simulink model "PI_observador_ideal_jhon"  (R2021b)
settings: Solver=VariableStepAuto  StartTime=0.0  StopTime=8  RelTol=1e-3
values from neighbouring files (symbols this model uses):
  K = [9.27647435897 40.5008113553]    [ValidarpiO.mat]
  ki = 111.439929309    [ValidarpiO.mat]
libraries: cstblocks x5
settings Model: Creator=axelt  LastModifiedBy=parra
settings DebuggingCC: UnconnectedInputMsg=none  UnconnectedOutputMsg=none  UnconnectedLineMsg=none
settings ModelReferenceCC: EnableRefExpFcnMdlSchedulingChecks=off
settings RTWCC: DLArmComputeVersion=20.02.1

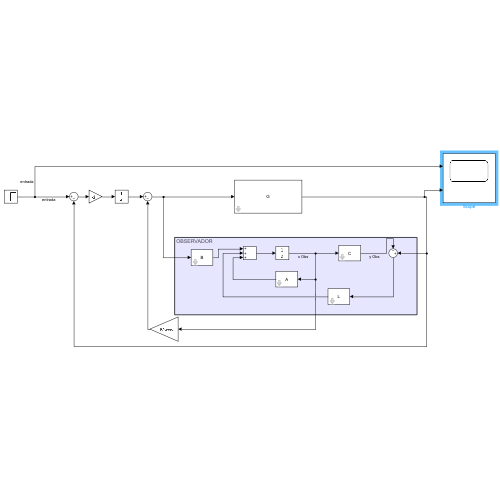
[thumbnail: Simulink's stored preview of the top-level diagram]
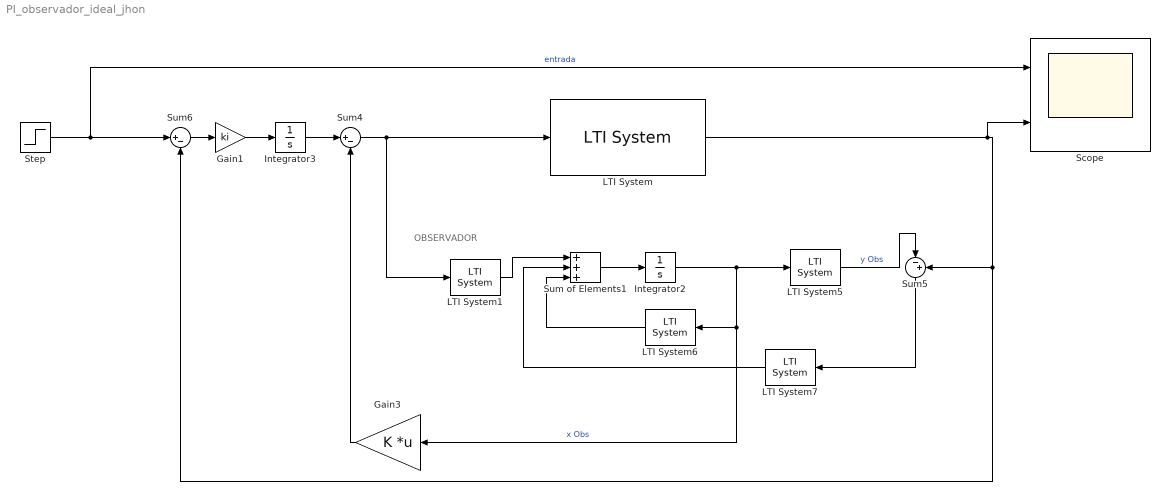
== system PI_observador_ideal_jhon ==
  note: OBSERVADOR
  Gain1 : Gain  Gain=ki
  Gain3 : Gain  Gain=K  Multiplication=Matrix(K*u) (u vector)
  Integrator2 : Integrator
  Integrator3 : Integrator
  LTI System : cstblocks/LTI System  sys=G  IC=[]
  LTI System1 : cstblocks/LTI System  sys=B  IC=[]
  LTI System5 : cstblocks/LTI System  sys=C  IC=[]
  LTI System6 : cstblocks/LTI System  sys=A  IC=[]
  LTI System7 : cstblocks/LTI System  sys=L  IC=[]
  Scope : Scope  NumInputPorts=2
  Step : Step  Time=4  Before=0.5  SampleTime=0.01
  Sum of Elements1 : Sum  Inputs=+++
  Sum4 : Sum  Inputs=|+-
  Sum5 : Sum  Inputs=|-+
  Sum6 : Sum  Inputs=|+-
  wires:
  Gain1/1 -> Integrator3/1
  Integrator3/1 -> Sum4/1
  Sum5/1 -> LTI System7/1
  Gain3/1 -> Sum4/2
  Integrator2/1 -> LTI System5/1, LTI System6/1, Gain3/1  "x Obs"
  Step/1 -> Scope/1, Sum6/1  "entrada"
  Sum4/1 -> LTI System/1, LTI System1/1
  LTI System1/1 -> Sum of Elements1/1
  LTI System6/1 -> Sum of Elements1/3
  Sum of Elements1/1 -> Integrator2/1
  LTI System5/1 -> Sum5/1  "y Obs"
  Sum6/1 -> Gain1/1
  LTI System7/1 -> Sum of Elements1/2
  LTI System/1 -> Scope/2, Sum5/2, Sum6/2
